simulink model "ncd_kalm_1"  (Simulink 4.00)
settings: Solver=ode45  StartTime=0.0  StopTime=50.0  RelTol=1e-3
values from neighbouring files (symbols this model uses):
  A = my_sys1.a    [ncd_estim1.m]    (also in ncd_estim_1.mat = [-0.48 2 0 0 0 0 -1.0376 0 1 0 0 0 ... (36 elements, 6x6)]; ncd_kalm1.m; ncd_kalm2.m; ncd_kalm_1.mat = [-0.48 2 0 0 0 0 -1.0376 0 1 0 0 0 ... (36 elements, 6x6)])
  B = my_sys1.b    [ncd_estim1.m]    (also in ncd_estim_1.mat = [0.5 0 0 0 0 0]; ncd_kalm1.m; ncd_kalm2.m; ncd_kalm_1.mat = [0.5 0 0 0 0 0])
  C = my_sys1.c    [ncd_estim1.m]    (also in ncd_estim_1.mat = [0 0 0 0 0 0.4608]; ncd_kalm1.m; ncd_kalm2.m; ncd_kalm_1.mat = [0 0 0 0 0 0.4608])
  D = my_sys1.d    [ncd_estim1.m]    (also in ncd_estim_1.mat = 0; ncd_kalm1.m; ncd_kalm2.m; ncd_kalm_1.mat = 0)
  ki = 1    [ncd_estim1.m]    (also in ncd_estim_1.mat = 1.82974576844; ncd_kalm1.m; ncd_kalm2.m; ncd_kalm_1.mat = 1.97821802246)
undefined symbols (not defined in the file or in its folder): ae, be
settings Model: LastModifiedBy=Administrator  BlockReductionOpt=off

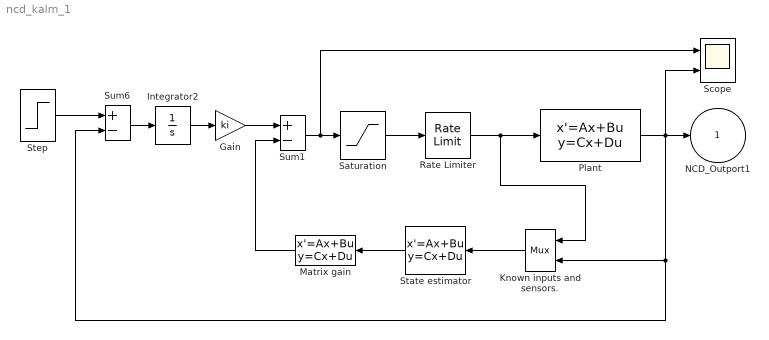
== system ncd_kalm_1 ==
  Gain : Gain  Gain=ki  Multiplication=Element-wise(K.*u)  SaturateOnIntegerOverflow=on
  Integrator2 : Integrator  ExternalReset=none  InitialConditionSource=internal  InitialCondition=0  LimitOutput=off  UpperSaturationLimit=inf  LowerSaturationLimit=-inf  ShowSaturationPort=off  ShowStatePort=off  AbsoluteTolerance=auto
  Known inputs and sensors. : Mux  Orientation=left  Inputs=[1,1]
      settings: DisplayOption=none
  Matrix gain : StateSpace  Orientation=left  A=[]  B=[]  C=[]  D=K  X0=0  Realization=auto  AbsoluteTolerance=auto  mask(Matrix gain){@1=[k1, k2, k3, k4, k5, k6]}
      mask prompts: @1 "Gain matrix:"
      mask help: Matrix Gain:
      mask init:
      | K = @1;
      mask Help: Multiplies input vector by entered matrix to produce output vector.
      mask Display: disp('K')
  Plant : StateSpace  A=A  B=B  C=C  D=D  X0=0  Realization=auto  AbsoluteTolerance=auto
  Rate Limiter : RateLimiter  RisingSlewLimit=10  FallingSlewLimit=-10
  Saturation : Saturate  UpperLimit=1  LowerLimit=-1  LinearizeAsGain=on
  Scope : Scope  NumInputPorts=2
      settings: TimeRange=auto  YMin=-5~-5  YMax=5~5  SaveToWorkspace=off  SaveName=ScopeData  LimitDataPoints=on  MaxDataPoints=5000
  State estimator : StateSpace  Orientation=left  A=ae  B=be  C=ce  D=de  X0=0  Realization=auto  AbsoluteTolerance=auto  mask(State estimator){@1=A, @2=B, @3=C, @4=D, @5=0.001*eye(ns,ns), @6=0.001}
      mask prompts: @1 "Plant A matrix:"; @2 "Plant B matrix:"; @3 "Plant C matrix:"; @4 "Plant D matrix:"; @5 "State noise covar. E[ww']:"; @6 "Output noise covar. E[vv']:"
      mask help:
      | Continuous Kalman state estimator.
      | (Requires Control Toolbox)
      mask init:
      | [nx,nu]=size(@2); [l,p]=lqe(@1,eye(nx,nx),@3,@5,@6); [ny,nx]=size(@3); [ae,be,cexy,dexy]=estim(@1,@2,@3,@4,l,1:ny,1:nu); ce=cexy(ny+1:ny+nx,:); de=dexy(ny+1:ny+nx,:);
      mask Help: Implements a Kalman state estimator using lqe and estim commands. Mask and unmask this block to see how it works.
      mask Display: disp('Kalman\nestimator')
  Step : Step  Time=0  Before=0  After=1  SampleTime=0
  Sum1 : Sum  Inputs=+-  SaturateOnIntegerOverflow=on
  Sum6 : Sum  Inputs=+-  SaturateOnIntegerOverflow=on
  NCD_Outport1 : Outport  Port=1  InitialOutput=0
      settings: OpenFcn=optblock
      mask Type: NCD Outport
      mask Display:
      | plot([0:10],[-.5 1.5 .6 1.3 .8 1.1 .95 1.02 .99 1 1]);
      | disp('\n\n NCD\n OutPort 1');
  wires:
  Gain/1 -> Sum1/1
  Matrix gain/1 -> Sum1/2
  Known inputs and sensors./1 -> State estimator/1
  State estimator/1 -> Matrix gain/1
  Rate Limiter/1 -> Plant/1, Known inputs and sensors./1
  Saturation/1 -> Rate Limiter/1
  Sum1/1 -> Saturation/1, Scope/1
  Step/1 -> Sum6/1
  Sum6/1 -> Integrator2/1
  Integrator2/1 -> Gain/1
  Plant/1 -> NCD_Outport1/1, Sum6/2, Known inputs and sensors./2, Scope/2
